simulink model "system_flowchart"  (R2024b)
settings: Solver=VariableStepAuto  StartTime=0.0  StopTime=10.0  RelTol=1e-3
settings Model: Creator=sahil  LastModifiedBy=sahil

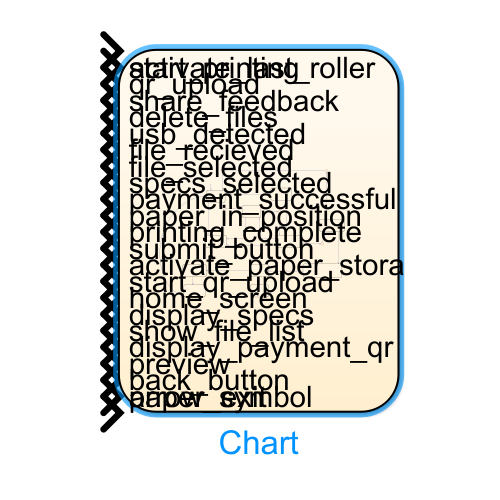
[thumbnail: Simulink's stored preview of the top-level diagram]
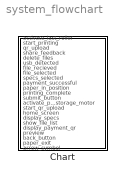
== system system_flowchart ==
  Chart : Stateflow chart  TreatAsAtomicUnit=on

== stateflow chart system_flowchart/Chart ==
  state FileUpload
    entry:
    start_qr_upload();
  state HomeScreen
    entry:
    home_screen();
  state print_preview
    entry:
    preview();
  state payment
    entry:
    display_payment_qr();
  state FileSelection
    entry:
    show_file_list();
  state SpecSelection
    entry:
    display_specs();
  state feedFromPaperStorage
    entry:
    activate_paper_storage_motor();
  state paperExit
    entry:
    activate_last_roller();
  state Printing
    entry:
    start_printing();
  state Feedback
    entry:
    share_feedback();
  state DeletionOfFiles
    entry:
    delete_files();
  (junction 90) -> (junction 92) : after(60,sec)
  (junction 92) -> HomeScreen
  payment -> (junction 90) [order 2]
  (default) -> HomeScreen
  HomeScreen -> FileUpload [order 1] : [qr_upload==1]
  Feedback -> HomeScreen : [submit_button==1 | after(10,sec)]
  FileUpload -> SpecSelection : [file_recieved==1]
  HomeScreen -> FileSelection [order 2] : [usb_detected==1]
  (junction 75) -> print_preview
  FileSelection -> (junction 75) : [file_selected==1]
  print_preview -> (junction 81) [order 1] : [arrow_symbol==1]
  (junction 81) -> SpecSelection
  print_preview -> (junction 77) [order 2] : [back_button==1]
  (junction 79) -> print_preview
  (junction 83) -> payment : [specs_selected==1]
  payment -> feedFromPaperStorage [order 1] : [payment_successful==1]
  (junction 77) -> FileSelection
  SpecSelection -> (junction 79) [order 3] : [arrow_symbol==0]
  SpecSelection -> (junction 83) [order 1]
  SpecSelection -> FileSelection [order 2] : [back_button==1]
  Printing -> paperExit [order 1] : [printing_complete==1]
  feedFromPaperStorage -> Printing : [paper_in_position==1]
  paperExit -> Feedback : [paper_exit==1]
  Printing -> DeletionOfFiles [order 2] : [printing_complete==1]
  data: activate_last_roller input; start_printing input; qr_upload input; share_feedback input; delete_files input; usb_detected input; file_recieved input; file_selected input; specs_selected input; payment_successful input; paper_in_position input; printing_complete input; submit_button input; activate_paper_storage_motor input; start_qr_upload input; home_screen input; display_specs input; show_file_list input; display_payment_qr input; preview input; back_button input; paper_exit input; arrow_symbol input
